simulink model "complete_fusion_system"  (R2022b)
settings: Solver=VariableStepAuto  StartTime=0.0  StopTime=45  FixedStep=t  RelTol=1e-3
values from neighbouring files (symbols this model uses):
  covA = 610    [fusion.m]    (also in fusion_parameters.m = 800; fusion_test.m = 0.00171675)
  covG = 0.76e-5    (= 7.6e-06)    [fusion.m]    (also in fusion_parameters.m = 0.0001; fusion_test.m = 0.004)
  covM = 0.4    [fusion.m]    (also in fusion_parameters.m = 80; fusion_test.m = 0)
  covP = 4    [fusion.m]    (also in fusion_parameters.m = 34; fusion_test.m = 0)
  covV = 0.01    [fusion.m]    (also in fusion_parameters.m = 0.0464; fusion_test.m = 0)
  fusion_t = 0.005    [fusion_parameters.m]
  gps_hz = 1/25    (= 0.04)    [fusion_parameters.m]
  imu_hz = 0.015    [fusion_parameters.m]
  IMUNED2VNED = rotmat(quaternion(IMU_ANGLE,"eulerd","XYZ","frame"),"frame")    [fusion_parameters.m]
  initstate = zeros(28,1)    [fusion_parameters.m]    (also in fusion_test.m)
  MAGNED2VNED = rotmat(quaternion(MAG_ANGLE,"eulerd","XYZ","frame"),"frame")    [fusion_parameters.m]
  ref_location = [40.437675, -86.943750, 680]    [fusion_parameters.m]
undefined symbols (not defined in the file or in its folder): sensor_angle
libraries: simulink x2, sensorgpslib x1, mspsensorlib x1
settings Model: Creator=fullb  LastModifiedBy=Inver

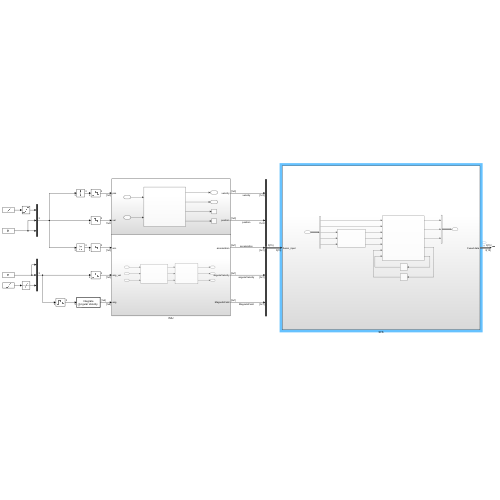
[thumbnail: Simulink's stored preview of the top-level diagram]
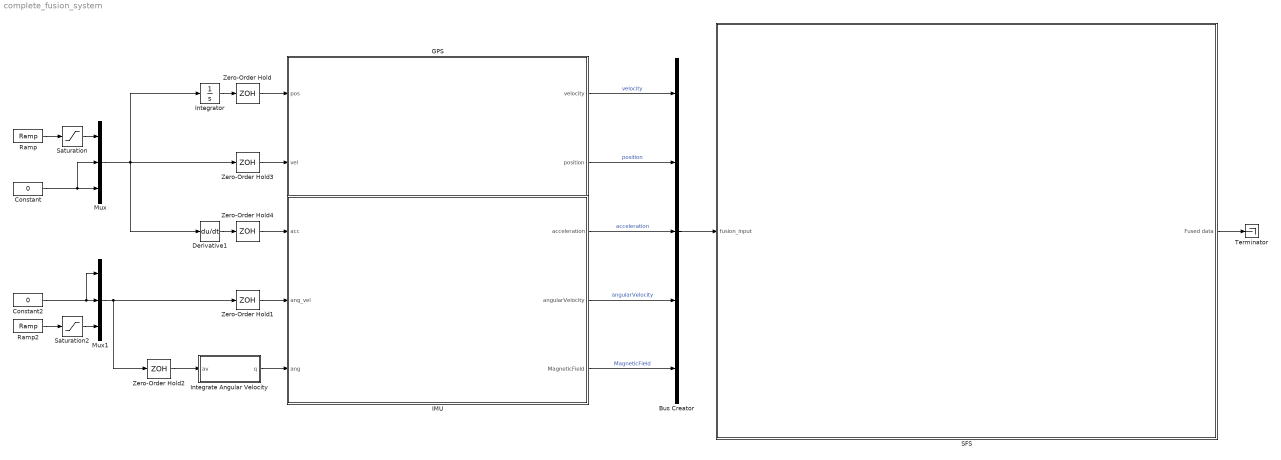
== system complete_fusion_system ==
  Bus Creator : BusCreator  Inputs=5
  Constant : Constant  Value=0
  Constant2 : Constant  Value=0
  Derivative1 : Derivative
  GPS : Subsystem
  IMU : Subsystem
  Integrate Angular Velocity : MATLAB Function  TreatAsAtomicUnit=on  mask{rate=imu_hz}
      mask prompts: rate "Sample Rate"
  Integrator : Integrator
  Mux : Mux  Inputs=3
  Mux1 : Mux  Inputs=3
  Ramp : simulink/Sources/Ramp  slope=3  start=0  InitialOutput=-30
  Ramp2 : simulink/Sources/Ramp  slope=1  start=0  InitialOutput=-20
  SFS : Subsystem
  Saturation : Saturate  UpperLimit=10  LowerLimit=0
  Saturation2 : Saturate  UpperLimit=2  LowerLimit=0
  Terminator : Terminator
  Zero-Order Hold : ZeroOrderHold  SampleTime=gps_hz
  Zero-Order Hold1 : ZeroOrderHold  SampleTime=imu_hz
  Zero-Order Hold2 : ZeroOrderHold  SampleTime=imu_hz
  Zero-Order Hold3 : ZeroOrderHold  SampleTime=gps_hz
  Zero-Order Hold4 : ZeroOrderHold  SampleTime=imu_hz
  wires:
  Bus Creator/1 -> SFS/1(fusion_input)
  SFS/1(Fused data) -> Terminator/1
  GPS/1(velocity) -> Bus Creator/1  "velocity"
  GPS/2(position) -> Bus Creator/2  "position"
  IMU/1(acceleration) -> Bus Creator/3  "acceleration"
  IMU/2(angularVelocity) -> Bus Creator/4  "angularVelocity"
  IMU/3(MagneticField) -> Bus Creator/5  "MagneticField"
  Mux/1 -> Zero-Order Hold3/1, Derivative1/1, Integrator/1
  Derivative1/1 -> Zero-Order Hold4/1
  Ramp/1 -> Saturation/1
  Constant/1 -> Mux/2, Mux/3
  Zero-Order Hold1/1 -> IMU/2(ang_vel)
  Zero-Order Hold2/1 -> Integrate Angular Velocity/1(av)
  Zero-Order Hold/1 -> GPS/1(pos)
  Zero-Order Hold3/1 -> GPS/2(vel)
  Zero-Order Hold4/1 -> IMU/1(acc)
  Integrator/1 -> Zero-Order Hold/1
  Saturation/1 -> Mux/1
  Constant2/1 -> Mux1/1, Mux1/2
  Saturation2/1 -> Mux1/3
  Ramp2/1 -> Saturation2/1
  Mux1/1 -> Zero-Order Hold2/1, Zero-Order Hold1/1
  Integrate Angular Velocity/1(q) -> IMU/3(ang)

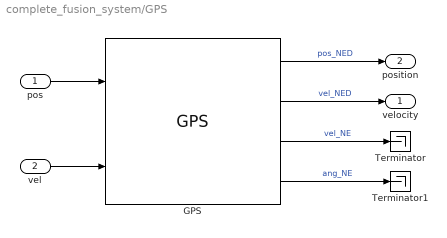
== system complete_fusion_system/GPS ==
  pos : Inport  PortDimensions=[1 3]
  vel : Inport  Port=2  PortDimensions=[1 3]
  GPS : sensorgpslib/GPS  DispRefFrame=NED  PositionInputFormat=Local  ReferenceLocation=ref_location  HorizontalPositionAccuracy=1.6  VerticalPositionAccuracy=3  VelocityAccuracy=0.1  DecayFactor=0.599  SeedDouble=67  SimulateUsing=Interpreted execution
      settings: LibrarySourceBlock=mspsensorlib/GPS
  Terminator : Terminator
  Terminator1 : Terminator
  velocity : Outport
  position : Outport  Port=2
  wires:
  GPS/1 -> position/1  "pos_NED"
  GPS/2 -> velocity/1  "vel_NED"
  GPS/3 -> Terminator/1  "vel_NE"
  GPS/4 -> Terminator1/1  "ang_NE"
  pos/1 -> GPS/1
  vel/1 -> GPS/2

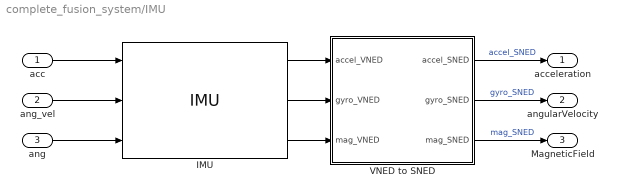
== system complete_fusion_system/IMU ==
  acc : Inport  PortDimensions=[1 3]
  ang_vel : Inport  Port=2  PortDimensions=[1 3]
  ang : Inport  Port=3  PortDimensions=[1 4]
  IMU : mspsensorlib/IMU  DispRefFrame=NED  Temperature=25  MagneticFieldNED=ref_mag_field  MagneticFieldENU=[ -2.4169, 27.5550, 16.0849 ]  SeedDouble=67  SimulateUsing=Interpreted execution  AccelParamsMeasurementRange=Inf  AccelParamsResolution=0  AccelParamsConstantBias=[ 0, 0, 0 ]  AccelParamsAxesMisalignment=[ 100, 0, 0; 0, 100, 0; 0, 0, 100 ]  AccelParamsNoiseDensity=[ 0, 0, 0 ]  AccelParamsBiasInstability=[ 0, 0, 0 ]  AccelParamsRandomWalk=[ 0, 0, 0 ]  AccelParamsTemperatureBias=[ 0, 0, 0 ]  AccelParamsTemperatureScaleFactor=[ 0, 0, 0 ]  GyroParamsMeasurementRange=Inf  GyroParamsResolution=0  GyroParamsConstantBias=[ 0, 0, 0 ]  GyroParamsAxesMisalignment=[ 100, 0, 0; 0, 100, 0; 0, 0, 100 ]  GyroParamsAccelerationBias=[ 0, 0, 0 ]  GyroParamsNoiseDensity=[ 0, 0, 0 ]  GyroParamsBiasInstability=[ 0, 0, 0 ]  GyroParamsRandomWalk=[ 0, 0, 0 ]  GyroParamsTemperatureBias=[ 0, 0, 0 ]  GyroParamsTemperatureScaleFactor=[ 0, 0, 0 ]  MagParamsMeasurementRange=Inf  MagParamsResolution=0  MagParamsConstantBias=[ 0, 0, 0 ]  MagParamsAxesMisalignment=[ 100, 0, 0; 0, 100, 0; 0, 0, 100 ]  MagParamsNoiseDensity=[ 0, 0, 0 ]  MagParamsBiasInstability=[ 0, 0, 0 ]  MagParamsRandomWalk=[ 0, 0, 0 ]  MagParamsTemperatureBias=[ 0, 0, 0 ]  MagParamsTemperatureScaleFactor=[ 0, 0, 0 ]
  VNED to SNED : MATLAB Function  TreatAsAtomicUnit=on
  acceleration : Outport
  angularVelocity : Outport  Port=2
  MagneticField : Outport  Port=3
  wires:
  IMU/1 -> VNED to SNED/1(accel_VNED)
  IMU/2 -> VNED to SNED/2(gyro_VNED)
  IMU/3 -> VNED to SNED/3(mag_VNED)
  ang_vel/1 -> IMU/2
  ang/1 -> IMU/3
  acc/1 -> IMU/1
  VNED to SNED/3(mag_SNED) -> MagneticField/1  "mag_SNED"
  VNED to SNED/2(gyro_SNED) -> angularVelocity/1  "gyro_SNED"
  VNED to SNED/1(accel_SNED) -> acceleration/1  "accel_SNED"

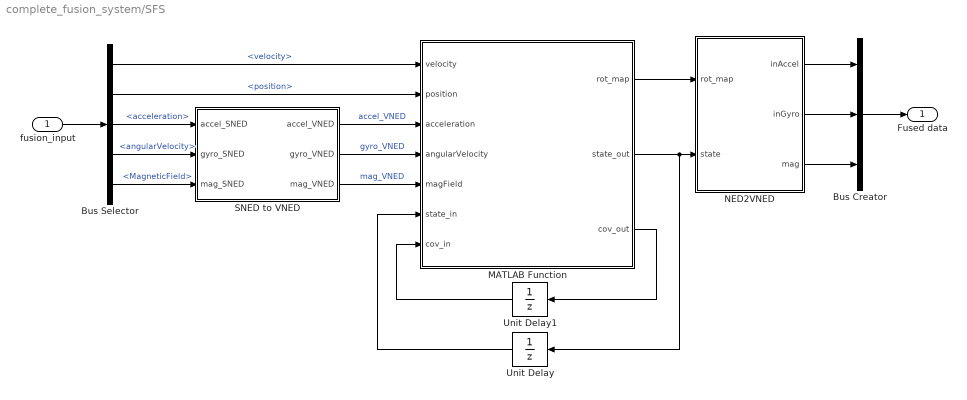
== system complete_fusion_system/SFS ==
  fusion_input : Inport
  Bus Creator : BusCreator  Inputs=3
  Bus Selector : BusSelector  OutputSignals=velocity,position,acceleration,angularVelocity,MagneticField
  MATLAB Function : MATLAB Function  TreatAsAtomicUnit=on  SystemSampleTime=fusion_t
  NED2VNED : MATLAB Function  TreatAsAtomicUnit=on
  SNED to VNED : MATLAB Function  TreatAsAtomicUnit=on  SystemSampleTime=fusion_t
  Unit Delay : UnitDelay  InitialCondition=initstate  SampleTime=fusion_t  HasFrameUpgradeWarning=on
  Unit Delay1 : UnitDelay  InitialCondition=eye(28)./1000  SampleTime=fusion_t  HasFrameUpgradeWarning=on
  Fused data : Outport
  wires:
  Bus Selector/1 -> MATLAB Function/1(velocity)  "<velocity>"
  Bus Selector/4 -> SNED to VNED/2(gyro_SNED)  "<angularVelocity>"
  Unit Delay/1 -> MATLAB Function/6(state_in)
  MATLAB Function/2(state_out) -> Unit Delay/1, NED2VNED/2(state)
  Bus Selector/2 -> MATLAB Function/2(position)  "<position>"
  Bus Selector/3 -> SNED to VNED/1(accel_SNED)  "<acceleration>"
  fusion_input/1 -> Bus Selector/1
  Bus Selector/5 -> SNED to VNED/3(mag_SNED)  "<MagneticField>"
  MATLAB Function/1(rot_map) -> NED2VNED/1(rot_map)
  Bus Creator/1 -> Fused data/1
  SNED to VNED/2(gyro_VNED) -> MATLAB Function/4(angularVelocity)  "gyro_VNED"
  SNED to VNED/1(accel_VNED) -> MATLAB Function/3(acceleration)  "accel_VNED"
  SNED to VNED/3(mag_VNED) -> MATLAB Function/5(magField)  "mag_VNED"
  MATLAB Function/3(cov_out) -> Unit Delay1/1
  Unit Delay1/1 -> MATLAB Function/7(cov_in)
  NED2VNED/1(inAccel) -> Bus Creator/1
  NED2VNED/2(inGyro) -> Bus Creator/2
  NED2VNED/3(mag) -> Bus Creator/3

== matlab function complete_fusion_system/Integrate Angular Velocity ==
  data: av input; q output; rate parameter
function q = integrateAngVel(av, rate)
%INTEGRATEANGVEL Integrate angular velocity to a quaternion
%  Treat Angular Velocity as an incremental rotation vector.

%   Copyright 2019 The MathWorks, Inc.   

persistent orient
if isempty(orient)
    % Initial orientation is the identity quaternion.
    orient = cast(quaternion(1,0,0,0), 'like', av);
end

% Convert angular velocity to a rotation vector.
rv = quaternion(av'*(rate), 'rotvec');
orient = rv * orient;
q = compact(orient);

== matlab function complete_fusion_system/SFS/MATLAB Function ==
  data: rot_map output; velocity input size=[1,3]; state_out output; position input size=[1,3]; acceleration input size=[1,3]; angularVelocity input size=[1,3]; magField input size=[1,3]; state_in input; cov_in input; covG parameter; covA parameter; covM parameter; covP parameter; covV parameter; fusion_t parameter; ref_location parameter; cov_out output
function [rot_map, state_out, cov_out] = fusion(velocity, position ,acceleration,angularVelocity, magField, state_in, cov_in, covG, covA, covM, covP, covV, fusion_t, ref_location) 

% creating the filter and loading previous state 
filter = insfilterAsync();
filter.ReferenceLocation = ref_location;
filter.State = state_in;
filter.StateCovariance = cov_in;

filter.AccelerationNoise = [1 1 1].*5;

% update filter state
predict(filter, fusion_t);

% Enforce Planar Conditions
position(3) = filter.ReferenceLocation(3);
velocity(3) = 0;

% the actual fusion
fuseaccel(filter,acceleration,covA);
fusegyro(filter,angularVelocity,covG);
fusemag(filter, magField,covM);
fusegps(filter,position,covP,velocity,covV);

[~,rot_map,~] = pose(filter, 'rotmat');

% Output matricies
state_out = filter.State;
cov_out = filter.StateCovariance;

end

== matlab function complete_fusion_system/SFS/NED2VNED ==
  data: rot_map input; state input; inAccel output; inGyro output; mag output
function [inAccel,inGyro, mag] = NED2VNED(rot_map,state)

orientation=state(1:4);
angvel=state(5:7);
pos=state(8:10);
vel=state(11:13);
accel=state(14:16);

%not sure which type frame/ point zyz/xyz etc...
% quat=quaternion(angles,"euler","XYZ","frame")
% rot_map=rotmat(quat,"frame")

%or inverse
inAccel= accel' * rot_map;
inGyro=rot_map;
mag=state(23:25);
end

== matlab function complete_fusion_system/IMU/VNED to SNED ==
  data: accel_SNED output; gyro_SNED output; accel_VNED input; gyro_VNED input; mag_VNED input; mag_SNED output; sensor_angle parameter; IMUNED2VNED parameter; MAGNED2VNED parameter
function [accel_SNED, gyro_SNED, mag_SNED] = VNED2SNED(accel_VNED, gyro_VNED, mag_VNED, sensor_angle, IMUNED2VNED, MAGNED2VNED)

% Construct Elemental Rotation Matrix
elemental_y = [cosd(sensor_angle) 0 sind(sensor_angle); 0 1 0; -sind(sensor_angle) 0 cosd(sensor_angle)];

% Rearrage matrix and compute elemental rotation
accel_SNED = elemental_y*[-accel_VNED(1); accel_VNED(2); -accel_VNED(3)];
gyro_SNED = elemental_y*[-gyro_VNED(1); gyro_VNED(2); -gyro_VNED(3)];
mag_SNED = elemental_y*[-mag_VNED(1); -mag_VNED(2); mag_VNED(3)];

== matlab function complete_fusion_system/SFS/SNED to VNED ==
  data: accel_VNED output size=[1 3]; gyro_VNED output size=[1 3]; accel_SNED input; gyro_SNED input; mag_SNED input; mag_VNED output size=[1 3]; sensor_angle parameter; IMUNED2VNED parameter; MAGNED2VNED parameter
function [accel_VNED, gyro_VNED, mag_VNED] = SNED2VNED(accel_SNED, gyro_SNED, mag_SNED, sensor_angle, IMUNED2VNED, MAGNED2VNED)

% Construct Elemental Rotation Matrix
elemental_y = [cosd(-sensor_angle) 0 sind(-sensor_angle); 0 1 0; -sind(-sensor_angle) 0 cosd(-sensor_angle)];

% Rearrage compute elemental rotation and rearrange matrix
accel_VNED = (elemental_y*accel_SNED)';
accel_VNED = [-accel_VNED(1) accel_VNED(2) -accel_VNED(3)];

gyro_VNED = (elemental_y*gyro_SNED)';
gyro_VNED = [-gyro_VNED(1) gyro_VNED(2) -gyro_VNED(3)];

mag_VNED = (elemental_y*mag_SNED)';
mag_VNED = [-mag_VNED(1) -mag_VNED(2) mag_VNED(3)];
